simulink model "chap5_8sim"  (Simulink 7.7)
settings: Solver=ode45  StartTime=0.0  StopTime=30  RelTol=1e-3
settings Model: Creator=Administrator  LastModifiedBy=ljk
settings DataIOCC: SignalLoggingName=sigsOut
settings OptimizationCC: InitFltsAndDblsToZero=on
settings DebuggingCC: SaveWithParameterizedLinksMsg=none  SignalResolutionControl=TryResolveAllWithWarning  SolverPrmCheckMsg=none  MultiTaskDSMMsg=warning  MultiTaskCondExecSysMsg=none  StrictBusMsg=None
settings HardwareCC: TargetUnknown=on
settings RTWCC: IncludeERTFirstTime=on
settings GRTTargetCC: TargetFcnLib=ansi_tfl_tmw.mat

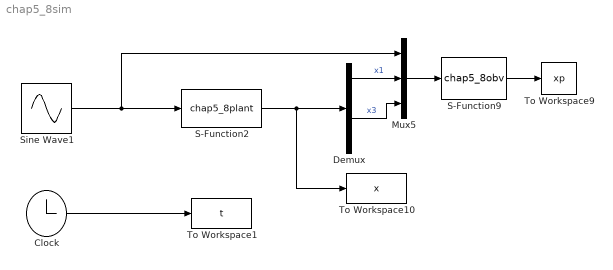
== system chap5_8sim ==
  Clock : Clock
      settings: Decimation=10
  Demux : Demux
  Mux5 : Mux  Inputs=3
  S-Function2 : S-Function  FunctionName=chap5_8plant  EnableBusSupport=off
  S-Function9 : S-Function  FunctionName=chap5_8obv  EnableBusSupport=off
  Sine Wave1 : Sin  SampleTime=0
  To Workspace1 : ToWorkspace  VariableName=t  SampleTime=-1  SaveFormat=Array
  To Workspace10 : ToWorkspace  VariableName=x  SampleTime=-1  SaveFormat=Array
  To Workspace9 : ToWorkspace  VariableName=xp  SampleTime=-1  SaveFormat=Array
  wires:
  Clock/1 -> To Workspace1/1
  Sine Wave1/1 -> S-Function2/1, Mux5/1
  S-Function2/1 -> To Workspace10/1, Demux/1
  Demux/1 -> Mux5/2  "x1"
  Demux/3 -> Mux5/3  "x3"
  Mux5/1 -> S-Function9/1
  S-Function9/1 -> To Workspace9/1
